simulink model "quadcopter_model"  (R2019a)
settings: Solver=FixedStepAuto  StartTime=0.0  StopTime=20  FixedStep=0.001  RelTol=1e-3
libraries: simulink x3, simulink_extras x1
settings Model: Creator=edoardo  LastModifiedBy=edoardo
settings OptimizationCC: DefaultParameterBehavior=Inlined  UseDivisionForNetSlopeComputation=on  GainParamInheritBuiltInType=on  UseFloatMulNetSlope=on  InlineInvariantSignals=on  PassReuseOutputArgsAs=Individual arguments  ZeroExternalMemoryAtStartup=off  ZeroInternalMemoryAtStartup=off  NoFixptDivByZeroProtection=on  EfficientFloat2IntCast=on  LifeSpan=1  OptimizeBlockOrder=speed  DifferentSizesBufferReuse=on
settings DebuggingCC: ParameterTunabilityLossMsg=error
settings HardwareCC: ProdBitPerPointer=32  ProdBitPerSizeT=32  ProdBitPerPtrDiffT=32  ProdLargestAtomicInteger=Long  ProdLargestAtomicFloat=Double  ProdWordSize=32  ProdLongLongMode=on  ProdHWDeviceType=ARM Compatible->ARM Cortex
settings SFSimCC: MATLABDynamicMemAlloc=off
settings RTWCC: SystemTargetFile=ert.tlc  TemplateMakefile=ert_default_tmf  GenerateReport=on  IncludeHyperlinkInReport=on  LaunchReport=on  GenerateTraceInfo=on  GenerateTraceReport=on  GenerateTraceReportSl=on  GenerateTraceReportSf=on  GenerateTraceReportEml=on  GenerateCodeMetricsReport=on
settings CodeAppCC: ForceParamTrailComments=on  IgnoreCustomStorageClasses=off  OperatorAnnotations=on  SimulinkDataObjDesc=on  SFDataObjDesc=on  CustomSymbolStrGlobalVar=rt$N$M  CustomSymbolStrType=$N$M  CustomSymbolStrFcn=$N$M$F  CustomSymbolStrMacro=$N$M  InsertBlockDesc=on
settings ERTTargetCC: TargetLangStandard=C99 (ISO)  GenerateSampleERTMain=on  IncludeMdlTerminateFcn=off  CombineSignalStateStructs=on  SupportAbsoluteTime=off  SupportComplex=off  SupportContinuousTime=on  SupportNonInlinedSFcns=on  InlinedParameterPlacement=NonHierarchical  ERTCustomFileTemplate=example_file_process.tlc  ERTFilePackagingFormat=CompactWithDataFile

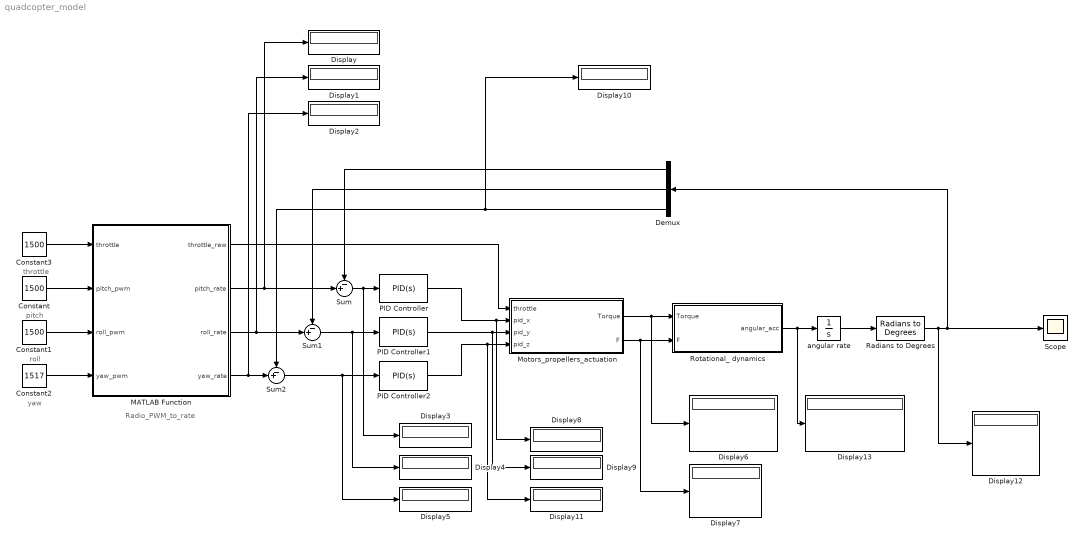
== system quadcopter_model ==
  note: Radio_PWM_to_rate
  note: throttle
  note: yaw
  note: roll
  note: pitch
  Constant : Constant  Value=1500
  Constant1 : Constant  Value=1500
  Constant2 : Constant  Value=1517
  Constant3 : Constant  Value=1500
  Demux : Demux  Outputs=3
  Display{,1..13} (14 alike) : Display
      Display6 settings: Decimation=2
  MATLAB Function : MATLAB Function  TreatAsAtomicUnit=on
  "Motors_propellers_actuation " : MATLAB Function  TreatAsAtomicUnit=on
  PID Controller : simulink/Continuous/PID Controller  Controller=PID  Form=Parallel  TimeDomain=Continuous-time  SampleTime=-1  IntegratorMethod=Forward Euler  FilterMethod=Forward Euler  ControllerParametersSource=internal  P=1.6  I=0  D=0  UseFilter=on  N=0  TunerSelectOption=Transfer Function Based (PID Tuner App)  ZeroCross=off  InitialConditionSource=internal  InitialConditionForIntegrator=0  InitialConditionForFilter=0  DifferentiatorICPrevScaledInput=0  ExternalReset=none  IgnoreLimit=on  TrackingMode=off  Kt=1  LimitOutput=on  UpperSaturationLimit=400  LowerSaturationLimit=-400  LinearizeAsGain=on  AntiWindupMode=clamping  Kb=1  POutMin=[]  POutMax=[]  IOutMin=[]  IOutMax=[]  DOutMin=[]  DOutMax=[]  NOutMin=[]  NOutMax=[]  SumOutMin=[]  SumOutMax=[]  SaturationOutMin=[]  SaturationOutMax=[]  PParamMin=[]  PParamMax=[]  IParamMin=[]  IParamMax=[]  DParamMin=[]  DParamMax=[]  NParamMin=[]  NParamMax=[]  KbParamMin=[]  KbParamMax=[]  KtParamMin=[]  KtParamMax=[]  KbOutMin=[]  KbOutMax=[]  KtOutMin=[]  KtOutMax=[]  IntegratorOutMin=[]  IntegratorOutMax=[]  FilterOutMin=[]  FilterOutMax=[]  SumI1OutMin=[]  SumI1OutMax=[]  SumI2OutMin=[]  SumI2OutMax=[]  SumI3OutMin=[]  SumI3OutMax=[]  SumI4OutMin=[]  SumI4OutMax=[]  SumDOutMin=[]  SumDOutMax=[]  DifferentiatorOutMin=[]  DifferentiatorOutMax=[]  FilterDiffOutCoefMin=[]  FilterDiffOutCoefMax=[]  ReciprocalOutMin=[]  ReciprocalOutMax=[]  SumDenOutMin=[]  SumDenOutMax=[]  SumNumOutMin=[]  SumNumOutMax=[]  DivideOutMin=[]  DivideOutMax=[]  IntegratorContinuousStateAttributes=''  IntegratorStateMustResolveToSignalObject=off  IntegratorRTWStateStorageClass=Auto  FilterContinuousStateAttributes=''  FilterStateMustResolveToSignalObject=off  FilterRTWStateStorageClass=Auto  ParallelPVariant=InternalParameters  IdealPVariant=Disabled  IVariant=InternalParameters  DVariant=InternalParameters  IntegratorVariant=Continuous  SatVariant=Enabled  AWVariant=ContClampingParallel  PCopyVariant=Disabled  TRVariant=Disabled  FdbkBlocksVariant=Forward  IdealPFdbkVariant=Disabled  SatFdbkVariant=Disabled  DerivativeFilterVariant=ContFilter  NVariant=InternalParameters  NCopyVariant=Disabled  FilterICVariant=InternalICsFilter  IntegratorICVariant=InternalICs  ExternalResetVariant=Disabled  TRSumVariant=Passthrough  SumFdbkVariant=Disabled  SumVariant=Sum_PID
  PID Controller1 : simulink/Continuous/PID Controller  Controller=PID  Form=Parallel  TimeDomain=Continuous-time  SampleTime=-1  IntegratorMethod=Forward Euler  FilterMethod=Forward Euler  ControllerParametersSource=internal  P=1.6  I=0  D=0  UseFilter=on  N=0  TunerSelectOption=Transfer Function Based (PID Tuner App)  InitialConditionSource=internal  InitialConditionForIntegrator=0  InitialConditionForFilter=0  DifferentiatorICPrevScaledInput=0  ExternalReset=none  IgnoreLimit=on  TrackingMode=off  Kt=1  LimitOutput=on  UpperSaturationLimit=400  LowerSaturationLimit=-400  LinearizeAsGain=on  AntiWindupMode=clamping  Kb=1  POutMin=[]  POutMax=[]  IOutMin=[]  IOutMax=[]  DOutMin=[]  DOutMax=[]  NOutMin=[]  NOutMax=[]  SumOutMin=[]  SumOutMax=[]  SaturationOutMin=[]  SaturationOutMax=[]  PParamMin=[]  PParamMax=[]  IParamMin=[]  IParamMax=[]  DParamMin=[]  DParamMax=[]  NParamMin=[]  NParamMax=[]  KbParamMin=[]  KbParamMax=[]  KtParamMin=[]  KtParamMax=[]  KbOutMin=[]  KbOutMax=[]  KtOutMin=[]  KtOutMax=[]  IntegratorOutMin=[]  IntegratorOutMax=[]  FilterOutMin=[]  FilterOutMax=[]  SumI1OutMin=[]  SumI1OutMax=[]  SumI2OutMin=[]  SumI2OutMax=[]  SumI3OutMin=[]  SumI3OutMax=[]  SumI4OutMin=[]  SumI4OutMax=[]  SumDOutMin=[]  SumDOutMax=[]  DifferentiatorOutMin=[]  DifferentiatorOutMax=[]  FilterDiffOutCoefMin=[]  FilterDiffOutCoefMax=[]  ReciprocalOutMin=[]  ReciprocalOutMax=[]  SumDenOutMin=[]  SumDenOutMax=[]  SumNumOutMin=[]  SumNumOutMax=[]  DivideOutMin=[]  DivideOutMax=[]  IntegratorContinuousStateAttributes=''  IntegratorStateMustResolveToSignalObject=off  IntegratorRTWStateStorageClass=Auto  FilterContinuousStateAttributes=''  FilterStateMustResolveToSignalObject=off  FilterRTWStateStorageClass=Auto  ParallelPVariant=InternalParameters  IdealPVariant=Disabled  IVariant=InternalParameters  DVariant=InternalParameters  IntegratorVariant=Continuous  SatVariant=Enabled  AWVariant=ContClampingParallel  PCopyVariant=Disabled  TRVariant=Disabled  FdbkBlocksVariant=Forward  IdealPFdbkVariant=Disabled  SatFdbkVariant=Disabled  DerivativeFilterVariant=ContFilter  NVariant=InternalParameters  NCopyVariant=Disabled  FilterICVariant=InternalICsFilter  IntegratorICVariant=InternalICs  ExternalResetVariant=Disabled  TRSumVariant=Passthrough  SumFdbkVariant=Disabled  SumVariant=Sum_PID
  PID Controller2 : simulink/Continuous/PID Controller  Controller=PID  Form=Parallel  TimeDomain=Continuous-time  SampleTime=-1  IntegratorMethod=Forward Euler  FilterMethod=Forward Euler  ControllerParametersSource=internal  P=3  I=0  D=0  UseFilter=on  N=0  TunerSelectOption=Transfer Function Based (PID Tuner App)  InitialConditionSource=internal  InitialConditionForIntegrator=0  InitialConditionForFilter=0  DifferentiatorICPrevScaledInput=0  ExternalReset=none  IgnoreLimit=on  TrackingMode=off  Kt=1  LimitOutput=on  UpperSaturationLimit=400  LowerSaturationLimit=-400  LinearizeAsGain=on  AntiWindupMode=clamping  Kb=1  POutMin=[]  POutMax=[]  IOutMin=[]  IOutMax=[]  DOutMin=[]  DOutMax=[]  NOutMin=[]  NOutMax=[]  SumOutMin=[]  SumOutMax=[]  SaturationOutMin=[]  SaturationOutMax=[]  PParamMin=[]  PParamMax=[]  IParamMin=[]  IParamMax=[]  DParamMin=[]  DParamMax=[]  NParamMin=[]  NParamMax=[]  KbParamMin=[]  KbParamMax=[]  KtParamMin=[]  KtParamMax=[]  KbOutMin=[]  KbOutMax=[]  KtOutMin=[]  KtOutMax=[]  IntegratorOutMin=[]  IntegratorOutMax=[]  FilterOutMin=[]  FilterOutMax=[]  SumI1OutMin=[]  SumI1OutMax=[]  SumI2OutMin=[]  SumI2OutMax=[]  SumI3OutMin=[]  SumI3OutMax=[]  SumI4OutMin=[]  SumI4OutMax=[]  SumDOutMin=[]  SumDOutMax=[]  DifferentiatorOutMin=[]  DifferentiatorOutMax=[]  FilterDiffOutCoefMin=[]  FilterDiffOutCoefMax=[]  ReciprocalOutMin=[]  ReciprocalOutMax=[]  SumDenOutMin=[]  SumDenOutMax=[]  SumNumOutMin=[]  SumNumOutMax=[]  DivideOutMin=[]  DivideOutMax=[]  IntegratorContinuousStateAttributes=''  IntegratorStateMustResolveToSignalObject=off  IntegratorRTWStateStorageClass=Auto  FilterContinuousStateAttributes=''  FilterStateMustResolveToSignalObject=off  FilterRTWStateStorageClass=Auto  ParallelPVariant=InternalParameters  IdealPVariant=Disabled  IVariant=InternalParameters  DVariant=InternalParameters  IntegratorVariant=Continuous  SatVariant=Enabled  AWVariant=ContClampingParallel  PCopyVariant=Disabled  TRVariant=Disabled  FdbkBlocksVariant=Forward  IdealPFdbkVariant=Disabled  SatFdbkVariant=Disabled  DerivativeFilterVariant=ContFilter  NVariant=InternalParameters  NCopyVariant=Disabled  FilterICVariant=InternalICsFilter  IntegratorICVariant=InternalICs  ExternalResetVariant=Disabled  TRSumVariant=Passthrough  SumFdbkVariant=Disabled  SumVariant=Sum_PID
  Radians to Degrees : simulink_extras/Transformations/Radians to Degrees
  "Rotational_ dynamics " : MATLAB Function  TreatAsAtomicUnit=on
  Scope : Scope
  Sum : Sum  Inputs=-+|
  Sum1 : Sum  Inputs=-+|
  Sum2 : Sum  Inputs=-+|
  angular rate : Integrator
  wires:
  Sum/1 -> Display3/1, PID Controller/1
  Sum1/1 -> Display4/1, PID Controller1/1
  Sum2/1 -> Display5/1, PID Controller2/1
  PID Controller/1 -> Display8/1, "Motors_propellers_actuation "/2(pid_x)
  PID Controller2/1 -> Display11/1, "Motors_propellers_actuation "/4(pid_z)
  PID Controller1/1 -> Display9/1, "Motors_propellers_actuation "/3(pid_y)
  "Motors_propellers_actuation "/1(Torque) -> Display6/1, "Rotational_ dynamics "/1(Torque)
  "Motors_propellers_actuation "/2(F) -> Display7/1, "Rotational_ dynamics "/2(F)
  "Rotational_ dynamics "/1(angular_acc) -> Display13/1, angular rate/1
  angular rate/1 -> Radians to Degrees/1
  Demux/1 -> Sum/1
  Demux/2 -> Sum1/1
  Demux/3 -> Display10/1, Sum2/1
  Radians to Degrees/1 -> Display12/1, Scope/1, Demux/1
  Constant3/1 -> MATLAB Function/1(throttle)
  MATLAB Function/1(throttle_raw) -> "Motors_propellers_actuation "/1(throttle)
  Constant/1 -> MATLAB Function/2(pitch_pwm)
  MATLAB Function/2(pitch_rate) -> Display/1, Sum/2
  Constant1/1 -> MATLAB Function/3(roll_pwm)
  MATLAB Function/3(roll_rate) -> Display1/1, Sum1/2
  Constant2/1 -> MATLAB Function/4(yaw_pwm)
  MATLAB Function/4(yaw_rate) -> Display2/1, Sum2/2

== matlab function quadcopter_model/Rotational_ dynamics  ==
  data: Torque input; angular_acc output; F input
function angular_acc = fcn(Torque, F)
    Moment      = [0 0 0];
    angular_acc = [0 0 0];
    Inertia     = [0.00305 0.00305 0.00611]; %Inertia for X,Y,Z
    axis_to_com = 0.1166;                    %distance between rotation axis and the center of mass of the vehicle

    
    Moment(1) = (F(1)+F(3))*axis_to_com-(F(2)+F(4))*axis_to_com;
    Moment(2) = (F(1)+F(2))*axis_to_com-(F(4)+F(3))*axis_to_com;
    Moment(3) = Torque(1)-Torque(2)-Torque(3)+Torque(4);
        
    for i = 1:3
        angular_acc(i) = Moment(i)/Inertia(i);
    end

end

== matlab function quadcopter_model/Motors_propellers_actuation  ==
  data: throttle input; pid_x input; Torque output; pid_y input; pid_z input; F output

function [Torque,F] = fcn(throttle,pid_x,pid_y,pid_z)
    %Parameters names, except the phisical ones, are directly taken from the C code implementation i.o.t. have 1:1 match  
    RPM            = [0 0 0 0];
    Torque         = [0 0 0 0];
    F              = [0 0 0 0];
    Voltage        = [0 0 0 0];
    
    if( throttle > 1800 )
        throttle = 1800;  %leave room for PID controller
    end
    
    Voltage(1) = throttle+pid_y+pid_x+pid_z;  %rear  right motor PWM
    Voltage(2) = throttle+pid_y-pid_x-pid_z;  %front right motor PWM
    Voltage(3) = throttle-pid_y+pid_x-pid_z;  %rear   left motor PWM
	Voltage(4) = throttle-pid_y-pid_x+pid_z;  %front  left motor PWM
   
    
    for i = 1:4     
        
        if(Voltage(i) > 2000)
            Voltage(i) = 2000;
        end
        
        if(Voltage(i) < 1100)
            Voltage(i) = 1100;
        end
        
        Voltage(i) = (Voltage(i)-1000)*0.0111;
        
        RPM(i)     = -1.87*Voltage(i)^3-1.08*10^-14*Voltage(i)^2+920*Voltage(i)-3.79*10^-14;
        Ct         = 6.3*10^-19*RPM(i)^4-1.51*10^-14*RPM(i)^3+1.21*10^-10*RPM(i)^2-2.58*10^-7*RPM(i)+0.12;
        F(i)       = Ct*1.225*(RPM(i)/60)^2*0.0017; % diam^4 = 0.001704
        %Torque(i)  = 5.19*10^-41*RPM(i)^10 - 5.63*10^-36*RPM(i)^9 + 2.27*10^-31*RPM(i)^8 - 4.63*10^-27*RPM(i)^7 + 5.21*10^-23*RPM(i)^6 - 3.16*10^-19*RPM(i)^5 + 7.77*10^-16*RPM(i)^4 + 1.37*10^-12*RPM(i)^3 -1.04*10^-8*RPM(i)^2 +1.68*10^-5*RPM(i) -9.22*10^-6;     
        Torque(i)  = -1.79*10^-26*RPM(i)^6+4.63*10^-21*RPM(i)^5-1.37*10^-16*RPM(i)^4+1.5*10^-12*RPM(i)^3-5.96*10^-9*RPM(i)^2+1.11*10^-5*RPM(i)+4.52*10^-4;     
    end

end

== matlab function quadcopter_model/MATLAB Function ==
  data: throttle input; throttle_raw output; pitch_pwm input; roll_pwm input; yaw_pwm input; pitch_rate output; roll_rate output; yaw_rate output
function [throttle_raw,pitch_rate,roll_rate,yaw_rate] = fcn(throttle,pitch_pwm,roll_pwm,yaw_pwm)

DEADBAND_UPPER_BOUND      = 1508;
DEADBAND_LOWER_BOUND      = 1492;
SETPOINT_PITCH_SPEED_RATE = 3.0;
SETPOINT_ROLL_SPEED_RATE  = 3.0;
SETPOINT_YAW_SPEED_RATE   = 3.0;

pitch_rate   = 0;
roll_rate    = 0;
yaw_rate     = 0;
throttle_raw = throttle;




if( pitch_pwm > DEADBAND_UPPER_BOUND )
    pitch_rate = ( pitch_pwm - DEADBAND_UPPER_BOUND ) / SETPOINT_PITCH_SPEED_RATE;
end
if( pitch_pwm < DEADBAND_LOWER_BOUND )
    pitch_rate = ( pitch_pwm - DEADBAND_LOWER_BOUND ) / SETPOINT_PITCH_SPEED_RATE;
end


if( roll_pwm > DEADBAND_UPPER_BOUND )
    roll_rate = ( roll_pwm - DEADBAND_UPPER_BOUND ) / SETPOINT_ROLL_SPEED_RATE;
end
if( pitch_pwm < DEADBAND_LOWER_BOUND )
    roll_rate = ( roll_pwm - DEADBAND_LOWER_BOUND ) / SETPOINT_ROLL_SPEED_RATE;
end


if( yaw_pwm > DEADBAND_UPPER_BOUND )
    yaw_rate = ( yaw_pwm - DEADBAND_UPPER_BOUND ) / SETPOINT_YAW_SPEED_RATE;
end
if( yaw_pwm < DEADBAND_LOWER_BOUND )
    yaw_rate = ( yaw_pwm - DEADBAND_LOWER_BOUND ) / SETPOINT_YAW_SPEED_RATE;
end


end
